simulink model "simulink_afbs_disturbance_rejection"  (Simulink 9.0)
settings: Solver=FixedStepAuto  StartTime=0.0  StopTime=simu.time  FixedStep=1e-5  RelTol=1e-4  EnableMultiTasking=on
values from neighbouring files (symbols this model uses):
  sys = tf(sys_zpk)    [main.m]    (also in main_compare_single_dual.m; main_cost_space.m; myFitness.m; myFitness_lamba_u.m)
undefined symbols (not defined in the file): afbs_params, taskset
settings Model: Creator=Xiaotian  LastModifiedBy=Steven
settings DataIOCC: LimitDataPoints=on
settings DebuggingCC: UnderspecifiedInitializationDetection=Simplified  MergeDetectMultiDrivingBlocksExec=error
settings GRTTargetCC: GeneratePreprocessorConditionals=Disable all

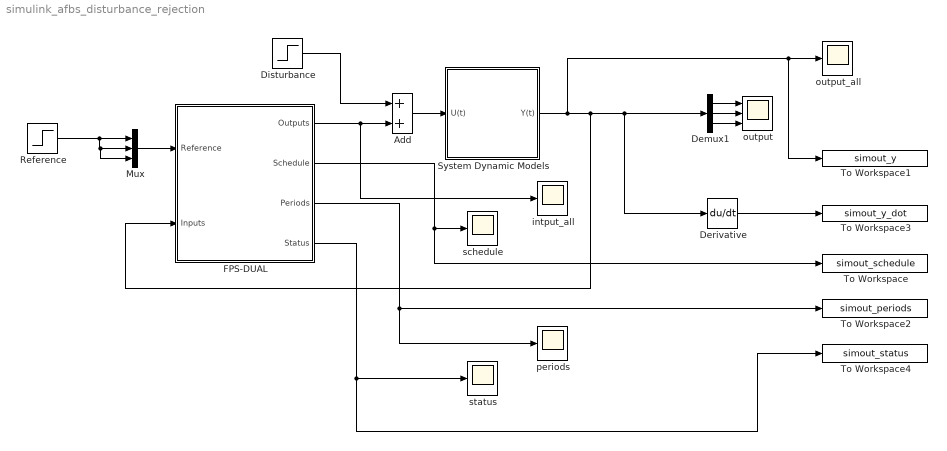
== system simulink_afbs_disturbance_rejection ==
  Add : Sum
  Demux1 : Demux  Outputs=3
  Derivative : Derivative
  Disturbance : Step  Time=0  After=0  SampleTime=0
  FPS-DUAL : Subsystem  mask{afbs_params__=afbs_params, task_params__=taskset}
      mask prompts: afbs_params__ "AFBS_Parameters"; task_params__ "Taskset"
      mask DialogControl DescTextVar Prompt: A Fixed-Priority Scheduler that supports adaptive and flexible scheduling.
  Mux : Mux  Inputs=3
  Reference : Step  Time=0  SampleTime=0
  System Dynamic Models : Subsystem
  To Workspace : ToWorkspace  VariableName=simout_schedule  SaveFormat=Timeseries  SampleTime=-1
  To Workspace1 : ToWorkspace  VariableName=simout_y  SaveFormat=Timeseries  SampleTime=-1
  To Workspace2 : ToWorkspace  VariableName=simout_periods  SaveFormat=Timeseries  SampleTime=-1
  To Workspace3 : ToWorkspace  VariableName=simout_y_dot  SaveFormat=Timeseries  SampleTime=-1
  To Workspace4 : ToWorkspace  VariableName=simout_status  SaveFormat=Timeseries  SampleTime=-1
  intput_all : Scope
  output : Scope  NumInputPorts=3
  output_all : Scope
  periods : Scope
  schedule : Scope
  status : Scope
  wires:
  FPS-DUAL/2(Schedule) -> To Workspace/1, schedule/1
  System Dynamic Models/1(Y(t)) -> FPS-DUAL/2(Inputs), Derivative/1, Demux1/1, output_all/1, To Workspace1/1
  Demux1/3 -> output/3
  Demux1/2 -> output/2
  Demux1/1 -> output/1
  FPS-DUAL/3(Periods) -> To Workspace2/1, periods/1
  Derivative/1 -> To Workspace3/1
  Reference/1 -> Mux/3, Mux/2, Mux/1
  Mux/1 -> FPS-DUAL/1(Reference)
  Disturbance/1 -> Add/1
  FPS-DUAL/1(Outputs) -> Add/2, intput_all/1
  Add/1 -> System Dynamic Models/1(U(t))
  FPS-DUAL/4(Status) -> status/1, To Workspace4/1

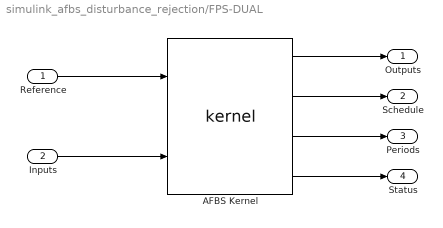
== system simulink_afbs_disturbance_rejection/FPS-DUAL ==
  Reference : Inport
  Inputs : Inport  Port=2
  AFBS Kernel : S-Function  FunctionName=kernel  Parameters=afbs_params__,task_params__  SFunctionDeploymentMode=off  EnableBusSupport=off
  Outputs : Outport
  Schedule : Outport  Port=2
  Periods : Outport  Port=3
  Status : Outport  Port=4
  wires:
  AFBS Kernel/1 -> Outputs/1
  AFBS Kernel/2 -> Schedule/1
  AFBS Kernel/3 -> Periods/1
  Reference/1 -> AFBS Kernel/1
  Inputs/1 -> AFBS Kernel/2
  AFBS Kernel/4 -> Status/1

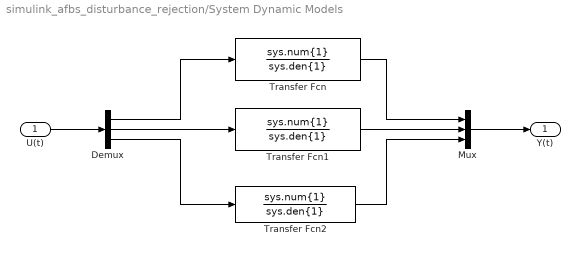
== system simulink_afbs_disturbance_rejection/System Dynamic Models ==
  U(t) : Inport
  Demux : Demux  Outputs=3
  Mux : Mux  Inputs=3
  Transfer Fcn : TransferFcn  Numerator=sys.num{1}  Denominator=sys.den{1}
  Transfer Fcn1 : TransferFcn  Numerator=sys.num{1}  Denominator=sys.den{1}
  Transfer Fcn2 : TransferFcn  Numerator=sys.num{1}  Denominator=sys.den{1}
  Y(t) : Outport
  wires:
  U(t)/1 -> Demux/1
  Demux/1 -> Transfer Fcn/1
  Demux/2 -> Transfer Fcn1/1
  Demux/3 -> Transfer Fcn2/1
  Transfer Fcn/1 -> Mux/1
  Transfer Fcn1/1 -> Mux/2
  Transfer Fcn2/1 -> Mux/3
  Mux/1 -> Y(t)/1
